simulink model "BLDC_DCTest"  (R2013a)
settings: Solver=ode45  StartTime=0.0  StopTime=10  RelTol=1e-3
libraries: powerlib x6
settings Model: Creator=Sony  LastModifiedBy=Muhammad Shamaas

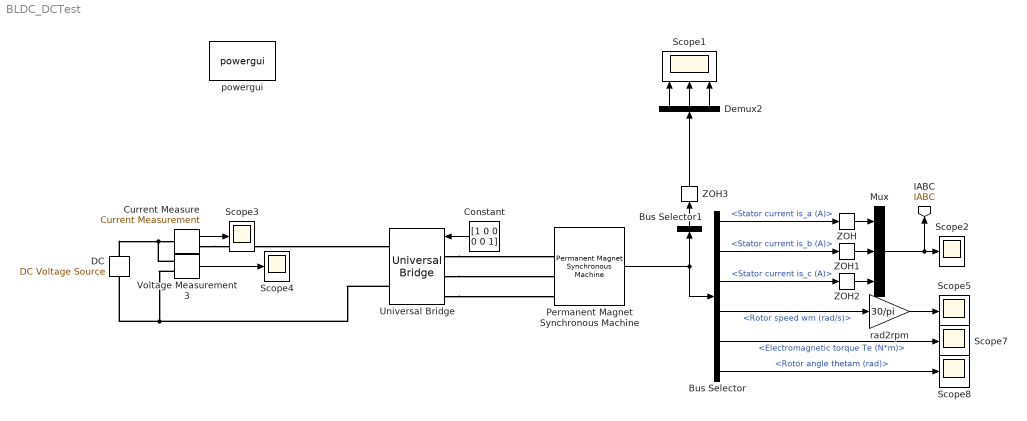
== system BLDC_DCTest ==
  Bus Selector : BusSelector  OutputSignals=Stator current is_a (A),Stator current is_b (A),Stator current is_c (A),Rotor speed wm (rad/s),Electromagnetic torque Te (N*m),Rotor angle thetam (rad)
  Bus Selector1 : BusSelector  OutputSignals=Hall effect signal h_a,Hall effect signal h_b,Hall effect signal h_c  OutputAsBus=on
  Constant : Constant  Value=[1 0 0 0 0 1]
  Current Measure : powerlib/Measurements/Current Measurement  PhasorSimulation=off  OutputType=Complex  PSBequivalent=0
  DC : powerlib/Electrical Sources/DC Voltage Source  Amplitude=1  Measurements=None
  Demux2 : Demux  Outputs=3
  Mux : Mux  Inputs=3
  Permanent Magnet Synchronous Machine : powerlib/Machines/Permanent Magnet Synchronous Machine  NbPhases=3  FluxDistribution=Trapezoidal  RotorType=Round  MechanicalLoad=Torque Tm  PresetModel=No  ShowDetailedParameters=on  Resistance=0.05  Inductance=1e-4  dqInductances=[8.5e-3,8.5e-3]  La=0.000835  MachineConstant=Torque Constant (N.m / A_peak)  Flux=0.0125  VoltageCst=10.472  TorqueCst=0.1  Flat=120  Mechanical=[ 1e-3, 1e-7 4]  PolePairs=4  InitialConditions=[(0)*(pi/30),0, 0,0]  InitialConditions5ph=[0 0 0 0 0 0]  TsPowergui=0  TsBlock=-1  RefAngle=Aligned with phase A axis (original Park)
  Scope1 : Scope  NumInputPorts=3
      settings: YMin=-1~-1~-1  YMax=2~2~2  SaveName=ScopeData3
  Scope{2..5,7..8} (6 alike) : Scope
      Scope2 settings: YMin=-250  YMax=250
      Scope3 settings: YMin=47.6  YMax=49.8
      Scope4 settings: YMin=-200  YMax=200  SaveName=ScopeData2
      Scope5 settings: YMin=0  YMax=5000  SaveName=ScopeData5
      Scope7 settings: YMin=0  YMax=70  SaveName=ScopeData9
      Scope8 settings: YMin=-0.139  YMax=-0.126  SaveName=ScopeData13
  Universal Bridge : powerlib/Power Electronics/Universal Bridge  Arms=3  SnubberResistance=1e5  SnubberCapacitance=inf  Device=MOSFET / Diodes  Ron=1e-3  Lon=0  ForwardVoltages="[  0  0  ]"  ForwardVoltage=0  GTOparameters=[ 10e-6 , 20e-6 ]  IGBTparameters=[ 1e-6 , 2e-6 ]  Measurements=None  Measurements_2=None  converterType=Rectifier
  Voltage Measurement3 : powerlib/Measurements/Voltage Measurement  PhasorSimulation=off  OutputType=Complex  PSBequivalent=0
  ZOH{,1..3} (4 alike) : ZeroOrderHold  SampleTime=1e-4
  powergui : powerlib/powergui  Priority=1  SimulationMode=Discrete  SolverType=Backward Euler  SampleTime=5e-5  frequency=60  SPID=off  DisableSnubberDevices=off  DisableRonSwitches=off  DisableVfSwitches=off  SwTol=0  Interpol=off  DisplayEquations=off  frequencyindice=0  Pbase=100e6  ErrMax=1e-4  Iterations=50  UnitsV=kV  UnitsW=MW  FunctionMessages=off  echomessages=off  HookPort=off  EnableUseOfTLC=off  x0status=blocks  RestoreLinks=warning  ResistiveCurrentMeasurement=off  Frange=[0:2:500]  Ylog=off  Xlog=on  ShowGrid=off  save=off  variable=ZData  ZoomFFT=off  StartTime=0.0  cycles=1  DisplayStyle=1  fundamental=60  FreqAxis=off  MaxFrequency=1000  frequencyindicesteady=1  RmsSteady=1  display=off  Ts=0  methode=off
  rad2rpm : Gain  Gain=30/pi
  tag scope: IABC=global
  wires:
  rad2rpm/1 -> Scope5/1
  Bus Selector/1 -> ZOH/1  "<Stator current is_a (A)>"
  Permanent Magnet Synchronous Machine/1 -> Bus Selector/1, Bus Selector1/1
  Bus Selector/2 -> ZOH1/1  "<Stator current is_b (A)>"
  Bus Selector/4 -> rad2rpm/1  "<Rotor speed wm (rad/s)>"
  Demux2/3 -> Scope1/3
  Demux2/2 -> Scope1/2
  Demux2/1 -> Scope1/1
  Bus Selector/3 -> ZOH2/1  "<Stator current is_c (A)>"
  Mux/1 -> Scope2/1, [IABC]
  ZOH/1 -> Mux/1
  ZOH1/1 -> Mux/2
  ZOH2/1 -> Mux/3
  Bus Selector1/1 -> ZOH3/1
  ZOH3/1 -> Demux2/1
  Current Measure/1 -> Scope3/1
  Voltage Measurement3/1 -> Scope4/1
  Bus Selector/5 -> Scope7/1  "<Electromagnetic torque Te (N*m)>"
  Bus Selector/6 -> Scope8/1  "<Rotor angle thetam (rad)>"
  Constant/1 -> Universal Bridge/1
  connections:
  DC/RConn1 -- Voltage Measurement3/LConn1 -- Current Measure/LConn1
  Voltage Measurement3/LConn2 -- DC/LConn1 -- Universal Bridge/RConn2
  Universal Bridge/LConn3 -- Permanent Magnet Synchronous Machine/LConn3
  Current Measure/RConn1 -- Universal Bridge/RConn1
  Universal Bridge/LConn1 -- Permanent Magnet Synchronous Machine/LConn1
  Universal Bridge/LConn2 -- Permanent Magnet Synchronous Machine/LConn2
